simulink model "sim_Exp81_part3"  (R2019a)
settings: Solver=VariableStepAuto  StartTime=0.0  StopTime=10.0  RelTol=1e-3
undefined symbols (not defined in the file): GP_den, GP_num, Kp_part1, L, T
settings Model: Creator=sgxgong4  LastModifiedBy=sgxgong4

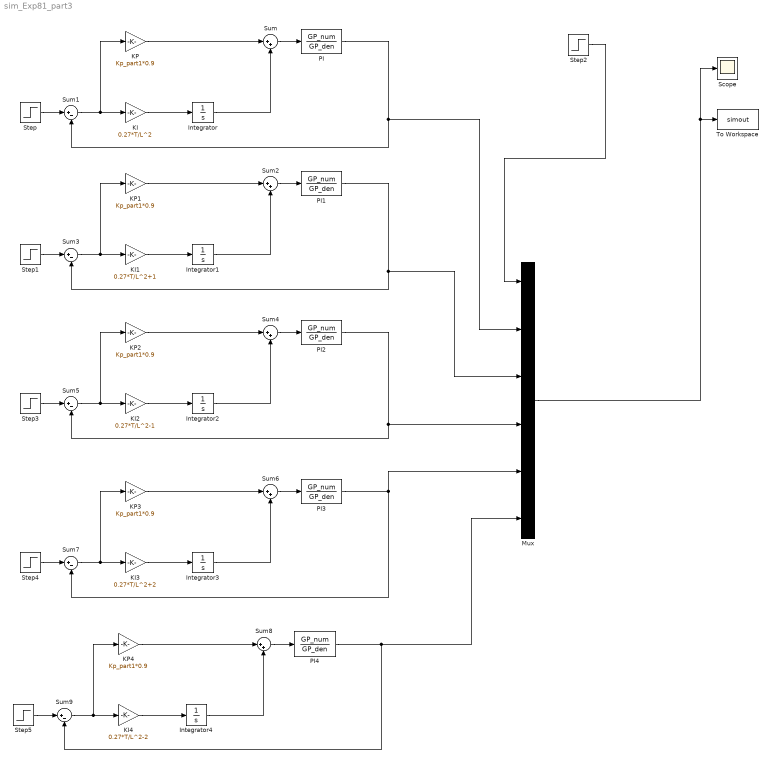
== system sim_Exp81_part3 ==
  Integrator{,1..4} (5 alike) : Integrator
  KI : Gain  Gain=0.27*T/L^2
  KI1 : Gain  Gain=0.27*T/L^2+1
  KI2 : Gain  Gain=0.27*T/L^2-1
  KI3 : Gain  Gain=0.27*T/L^2+2
  KI4 : Gain  Gain=0.27*T/L^2-2
  KP{,1..4} (5 alike) : Gain  Gain=Kp_part1*0.9
  Mux : Mux  Inputs=6
  PI{,1..4} (5 alike) : TransferFcn  Numerator=GP_num  Denominator=GP_den
  Scope : Scope
  Step{,1..5} (6 alike) : Step  Time=0  SampleTime=0
  Sum{,2,4,6,8} (5 alike) : Sum  Inputs=|++
  Sum{1,3,5,7,9} (5 alike) : Sum  Inputs=|+-
  To Workspace : ToWorkspace  VariableName=simout  SaveFormat=Structure With Time  SampleTime=-1
  wires:
  KI/1 -> Integrator/1
  KP/1 -> Sum/1
  Integrator/1 -> Sum/2
  Sum1/1 -> KP/1, KI/1
  Step/1 -> Sum1/1
  Sum/1 -> PI/1
  PI/1 -> Sum1/2, Mux/2
  Mux/1 -> To Workspace/1, Scope/1
  Step2/1 -> Mux/1
  Integrator1/1 -> Sum2/2
  PI1/1 -> Mux/3, Sum3/2
  Sum2/1 -> PI1/1
  Step1/1 -> Sum3/1
  Sum3/1 -> KP1/1, KI1/1
  KI1/1 -> Integrator1/1
  KP1/1 -> Sum2/1
  Integrator2/1 -> Sum4/2
  PI2/1 -> Sum5/2, Mux/4
  Sum4/1 -> PI2/1
  Step3/1 -> Sum5/1
  Sum5/1 -> KP2/1, KI2/1
  KI2/1 -> Integrator2/1
  KP2/1 -> Sum4/1
  Integrator3/1 -> Sum6/2
  PI3/1 -> Sum7/2, Mux/5
  Sum6/1 -> PI3/1
  Step4/1 -> Sum7/1
  Sum7/1 -> KP3/1, KI3/1
  KI3/1 -> Integrator3/1
  KP3/1 -> Sum6/1
  Integrator4/1 -> Sum8/2
  PI4/1 -> Sum9/2, Mux/6
  Sum8/1 -> PI4/1
  Step5/1 -> Sum9/1
  Sum9/1 -> KP4/1, KI4/1
  KI4/1 -> Integrator4/1
  KP4/1 -> Sum8/1
